simulink model "VCU_Top_Level"  (R2023b)
settings: Solver=VariableStepAuto  StartTime=0.0  StopTime=20  RelTol=1e-3
settings Model: Creator=heyka  LastModifiedBy=diego
settings DebuggingCC: UnconnectedInputMsg=warning  UnconnectedOutputMsg=warning  UnconnectedLineMsg=warning
settings ModelReferenceCC: EnableRefExpFcnMdlSchedulingChecks=on
settings RTWCC: DLArmComputeVersion=19.05

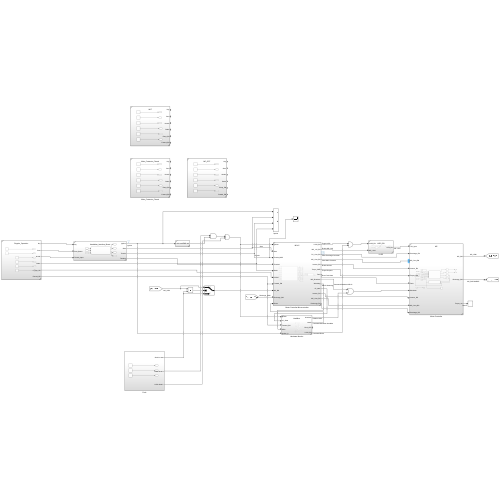
[thumbnail: Simulink's stored preview of the top-level diagram]
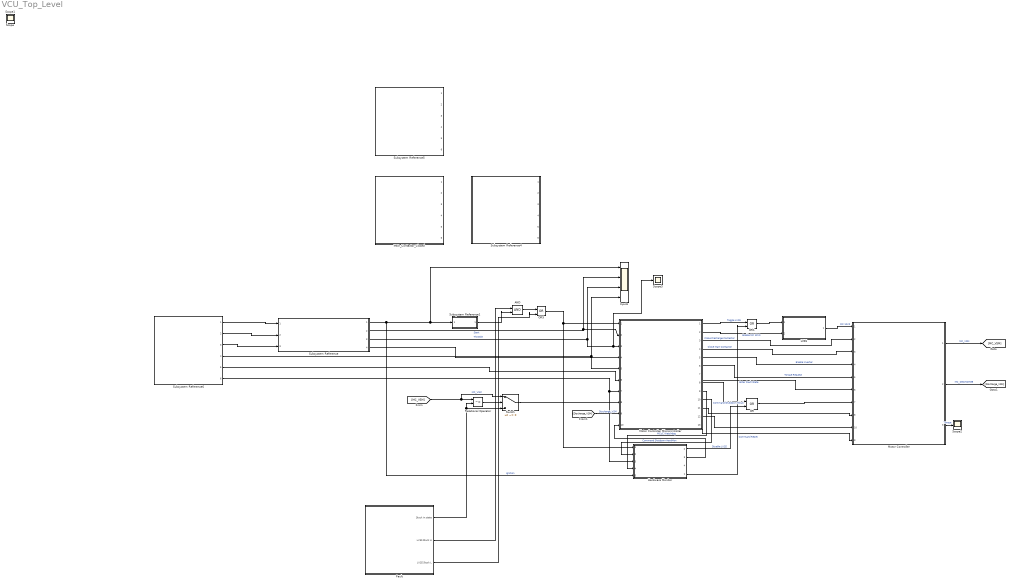
== system VCU_Top_Level ==
  AND : Logic  IconShape=distinctive  AllPortsSameDT=off  OutDataTypeStr=boolean
  Fault : Subsystem
  Hardware Monitor : Subsystem  ReferencedSubsystem=HardMon
      settings: PortSchema="{\"entries\":[{\"content\":{\"sides\":[{\"content\":{\"connectorIds\":[\"In1\",\"In2\",\"In3\",\"In4\",\"In5\"]},\"type\":\"ConnectorPlacement.EquallySpacedRectSide\",\"uuid\":\"af5c6d9c-e8dd-437b-8525-b8b1b8078e7c\"},{\"content\":{\"connectorIds\":[\"Out2\",\"Out3\",\"Out4\",\"Out1\"],\"side\":\"RIGHT\"},\"type\":\"ConnectorPlacement.EquallySpacedRectSide\",\"uuid\":\"28a6eb99-52ec-446a-9d54-51afb1295ac0\"},{\"content\":{\"side\":\"TOP\"},\"type\":\"ConnectorPlacement.EquallySpacedRectSide\",\"uuid\":\"7799cb04-bb33-48e0-a4da-089a7c648667\"}]},\"type\":\"ConnectorPlacement.EquallySpacedConnector\",\"uuid\":\"4e465d29-5fe7-4910-8123-a7e02f463998\"}],\"packageUris\":[\"http://schema.mathworks.com/mf0/Connector/R2020b\"],\"version\":\"1.0\"}"
  Inputs : Scope  NumInputPorts=4
  LVSS : Subsystem  ReferencedSubsystem=LVSS_EN
  Main_Contactor_Closed : Subsystem  ReferencedSubsystem=Main_Contactor_Closed
  Motor Controller : Subsystem  ReferencedSubsystem=MC
      settings: PortSchema="{\"entries\":[{\"content\":{\"sides\":[{\"content\":{\"connectorIds\":[\"In1\",\"In2\",\"In3\",\"In4\",\"In5\",\"In6\",\"In7\",\"In8\",\"In10\",\"In9\"]},\"type\":\"ConnectorPlacement.EquallySpacedRectSide\",\"uuid\":\"a8f99348-1313-4974-b079-6519fae7d892\"},{\"content\":{\"connectorIds\":[\"Out1\",\"Out2\",\"Out3\"],\"side\":\"RIGHT\"},\"type\":\"ConnectorPlacement.EquallySpacedRectSide\",\"uuid\":\"8c11e382-97e6-4294-8c7e-77f45cf735ae\"},{\"content\":{\"side\":\"TOP\"},\"type\":\"ConnectorPlacement.EquallySpacedRectSide\",\"uuid\":\"c9745617-8187-432a-91b2-b5ea6180bd92\"}]},\"type\":\"ConnectorPlacement.EquallySpacedConnector\",\"uuid\":\"0eb1e3ce-728a-4850-b2f6-0ae879968050\"}],\"packageUris\":[\"http://schema.mathworks.com/mf0/Connector/R2020b\"],\"version\":\"1.0\"}"
  Motor Controller Microcontroller : Subsystem  ReferencedSubsystem=MCuC
  OR : Logic  Operator=OR  IconShape=distinctive  AllPortsSameDT=off  OutDataTypeStr=boolean
  OR1 : Logic  Operator=OR  IconShape=distinctive  AllPortsSameDT=off  OutDataTypeStr=boolean
  OR5 : Logic  Operator=OR  IconShape=distinctive  AllPortsSameDT=off  OutDataTypeStr=boolean
  Relational Operator : RelationalOperator  Operator=~=  OutDataTypeStr=boolean  RndMeth=Simplest  InputSameDT=off
  Scope{,1..3} (4 alike) : Scope
  Subsystem Reference : Subsystem  ReferencedSubsystem=Handlebar_Interface_Board
  Subsystem Reference1 : Subsystem  ReferencedSubsystem=LevelShift
  Subsystem Reference4 : Subsystem  ReferencedSubsystem=MC_OFF
  Subsystem Reference5 : Subsystem  ReferencedSubsystem=INIT
  Subsystem Reference6 : Subsystem  ReferencedSubsystem=Regular_Operation
  Switch : Switch  Criteria=u2 ~= 0  Threshold=3  SaturateOnIntegerOverflow=off  InputSameDT=off
  wires:
  Subsystem Reference6/2 -> Subsystem Reference/2
  Motor Controller Microcontroller/4 -> Motor Controller/3  "Close Main Contactor"
  OR/1 -> Motor Controller/7
  Subsystem Reference/3 -> Inputs/3, Scope3/1, Motor Controller Microcontroller/3  "Throttle"
  Motor Controller Microcontroller/2 -> LVSS/2  "Enable MC 12V0"
  Subsystem Reference6/4 -> Inputs/4, Motor Controller Microcontroller/5
  [Discharge_VSM] -> Motor Controller Microcontroller/9  "Discharge_VSM"
  Motor Controller Microcontroller/6 -> Motor Controller/5  "Torque Request"
  Subsystem Reference/2 -> Motor Controller Microcontroller/2, Inputs/2  "Start"
  Motor Controller/1 -> [MC_VSM]  "MC_VSM"
  Motor Controller/2 -> [Discharge_VSM]  "MC_DISCHARGE"
  Subsystem Reference6/1 -> Subsystem Reference/1
  Subsystem Reference/1 -> Hardware Monitor/5, Inputs/1, Subsystem Reference1/1  "Ignition"
  Motor Controller Microcontroller/1 -> OR1/1  "Toggle LVSS"
  LVSS/1 -> Motor Controller/1  "MC 12V0"
  Motor Controller Microcontroller/7 -> Motor Controller/6  "Enter Fault State"
  Subsystem Reference6/3 -> Subsystem Reference/3
  Motor Controller Microcontroller/3 -> Motor Controller/2  "Close Precharge Contactor"
  Subsystem Reference6/6 -> Hardware Monitor/3, Motor Controller Microcontroller/7
  Motor Controller Microcontroller/5 -> Motor Controller/4  "Enable Inverter"
  OR1/1 -> LVSS/1
  Motor Controller Microcontroller/11 -> Motor Controller/8
  Motor Controller Microcontroller/13 -> Motor Controller/9
  Motor Controller Microcontroller/12 -> Motor Controller/10
  Motor Controller Microcontroller/8 -> OR/1  "Command Shutdown MCuC"
  Motor Controller/3 -> Scope2/1  "Torque"
  Subsystem Reference/4 -> Motor Controller Microcontroller/4
  [MC_VSM] -> Relational Operator/1, Switch/1  "MC_VSM"
  Switch/1 -> Motor Controller Microcontroller/8
  Relational Operator/1 -> Switch/2
  Fault/1(Stuck in state) -> Switch/3, Relational Operator/2
  Hardware Monitor/2 -> OR/2  "Disable LVSS"
  Hardware Monitor/3 -> Motor Controller Microcontroller/10  "Command Shutdown HardMon"
  Hardware Monitor/1 -> OR1/2  "Command Reset"
  Motor Controller Microcontroller/9 -> Hardware Monitor/4  "MCuC Watchdog"
  Motor Controller Microcontroller/10 -> Hardware Monitor/2
  Subsystem Reference6/5 -> Motor Controller Microcontroller/6
  Subsystem Reference1/1 -> AND/2
  Fault/2(LVSS Stuck H) -> AND/1
  OR5/1 -> Hardware Monitor/1, Motor Controller Microcontroller/1
  AND/1 -> OR5/1
  Fault/3(LVSS Stuck L) -> OR5/2

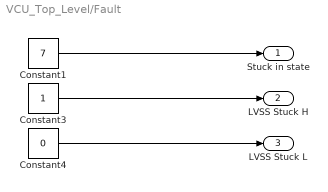
== system VCU_Top_Level/Fault ==
  Constant1 : Constant  Value=7
  Constant3 : Constant
  Constant4 : Constant  Value=0
  Stuck in state : Outport
  LVSS Stuck H : Outport  Port=2
  LVSS Stuck L : Outport  Port=3
  wires:
  Constant1/1 -> Stuck in state/1
  Constant3/1 -> LVSS Stuck H/1
  Constant4/1 -> LVSS Stuck L/1
